simulink model "toPWM"  (R2015b)
settings: Solver=VariableStepAuto  StartTime=0.0  StopTime=inf  RelTol=1e-3
undefined symbols (not defined in the file or in its folder): Controls, GroupMix
libraries: robotlib x2
settings Model: Creator=erik  LastModifiedBy=rasrack

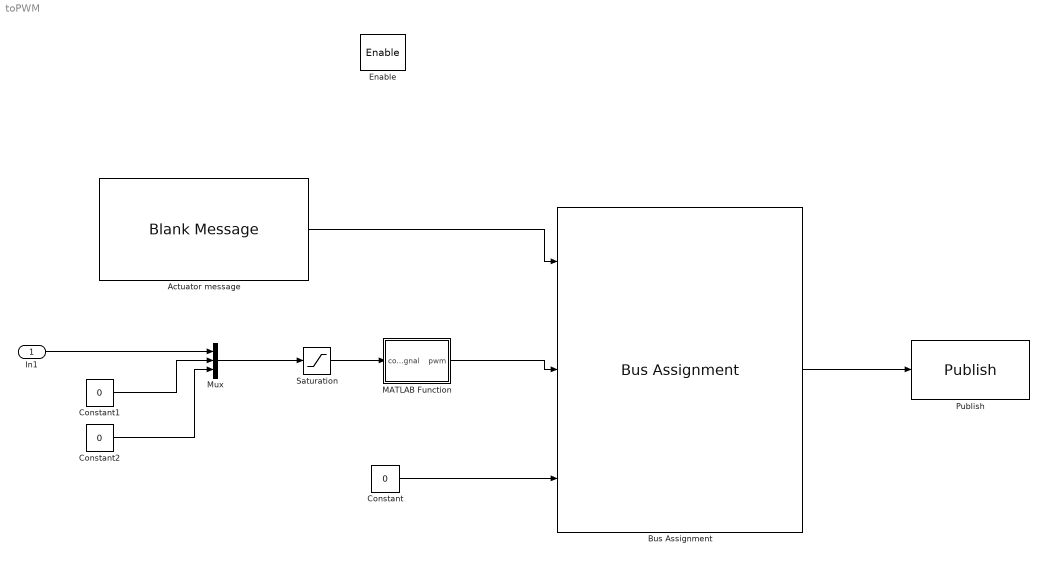
== system toPWM ==
  In1 : Inport  OutDataTypeStr=single  PortDimensions=6
  Enable : EnablePort
  "Actuator message " : robotlib/Blank Message  SourceLibraryInfo=This block requires Robotics System Toolbox  messageType=mavros_msgs/ActuatorControl  SampleTime=inf
  Bus Assignment : BusAssignment  AssignedSignals=Controls,GroupMix
  Constant : Constant  Value=0  OutDataTypeStr=uint8
  Constant1 : Constant  Value=0  OutDataTypeStr=single
  Constant2 : Constant  Value=0  OutDataTypeStr=single
  MATLAB Function : MATLAB Function  TreatAsAtomicUnit=on
  Mux : Mux  Inputs=3
  Publish : robotlib/Publish  SourceLibraryInfo=This block requires Robotics System Toolbox  topicSource=Select from ROS network  topic=/mavros/actuator_control  messageType=mavros_msgs/ActuatorControl  messageQueueLength=1
  Saturation : Saturate  UpperLimit=1  LowerLimit=-1
  wires:
  "Actuator message "/1 -> Bus Assignment/1
  Constant/1 -> Bus Assignment/3
  Bus Assignment/1 -> Publish/1
  MATLAB Function/1(pwm) -> Bus Assignment/2
  Saturation/1 -> MATLAB Function/1(controlsignal)
  In1/1 -> Mux/1
  Constant1/1 -> Mux/2
  Constant2/1 -> Mux/3
  Mux/1 -> Saturation/1

== matlab function toPWM/MATLAB Function ==
  data: controlsignal input; pwm output
function pwm = calcPWM(controlsignal)
 % thruster values should be between 1100 and 1900 microseconds (us)
 % values less than 1500 us are backwards; values more than are forwards

pwm=(controlsignal + 1) * 400 + 1100;

end
